simulink model "flightControlSystem"  (R2024b)
settings: Solver=ode3  StartTime=0  StopTime=TFinal  FixedStep=Ts  RelTol=1e-3  EnableMultiTasking=on
undefined symbols (not defined in the file): BINARIZER_THRESHOLD, codertarget, COG_X, COG_Xe, COG_Y, COG_Ye, Controller, DELAY_LANDING, DERIVATIVE_GAIN_X, DERIVATIVE_GAIN_Y, DiscIntNeverNeededParam, Discrete, DISK_KERNEL, Estimator, FLAG_WAIT_FOR_HOVERING, FOV, FOV_inner, FRAME_SIZE_HEIGHT, FRAME_SIZE_WIDTH, g, GAIN_LANDING, GAIN_TRACK, gray, init, MAX_RADIUS_CROWN, MAX_RADIUS_TRACK, MIN_RADIUS_CROWN, MIN_RADIUS_TRACK, Sensors, SQUARE_KERNEL, strel, Time, TIME_HOLD_X, TIME_HOLD_Y, Ts, var_acc_angle_N, var_bias_gyr_N, var_gyro_p_N, Vehicle, Z_HIGH, Z_LOW
libraries: simulink x39, slpidlib x4, ctrlSharedLib x4, sharedtransform x3, visionmorphops x2, parrotlib x1
(part 3 of 3)

== matlab function flightControlSystem/Image Processing System/MATLAB Function1 ==
  data: binary input; error_x_end_marker output; waypoint_follower_variable input; FRAME_SIZE_WIDTH input; FRAME_SIZE_HEIGHT input; COG_Y input; COG_X input; error_y_end_marker output; flag_end_marker output
function [error_x_end_marker, error_y_end_marker, flag_end_marker] = end_marker_detector(binary, waypoint_follower_variable, ...
    FRAME_SIZE_WIDTH, FRAME_SIZE_HEIGHT, COG_Y, COG_X)


persistent column_accumulator
persistent count_pixel
persistent row_accumulator

if isempty(column_accumulator)
    column_accumulator = 0;
end

if isempty(count_pixel)
    count_pixel = 0;
end

if isempty(row_accumulator)
    row_accumulator = 0;
end

flag_track = waypoint_follower_variable(3);

% check if the track is ended
if ~flag_track

    for i=1:FRAME_SIZE_HEIGHT

        for j=1:FRAME_SIZE_WIDTH

            %check all the pixel belonging to the end marker
            if binary(i,j)==1
                count_pixel = count_pixel +1;
                column_accumulator = column_accumulator + j;
                row_accumulator = row_accumulator + i;

            end

        end
    end
    
    if count_pixel ~= 0
        flag_end_marker=1;
        center_x = round(row_accumulator/count_pixel);
        center_y = round(column_accumulator/count_pixel);
    else
        flag_end_marker=0;              %for last push to the landing location
        center_x=0;
        center_y=0;
    end

else
    
    center_x = 0;
    center_y = 0;
    flag_end_marker = 0;

end

% Calculate the medium point of the end marker
error_x_end_marker = -(center_x - COG_X);
error_y_end_marker = (center_y - COG_Y);

% reset of the persistent variables
count_pixel = 0;
column_accumulator = 0;
row_accumulator = 0;

end

== stateflow chart flightControlSystem/Control System/Path Planning/Chart ==
  state State0
    during:
    x_error = 0;
    y_error = 0;
  state State2
    during:
    x_error = x_err_tr;
    y_error = y_err_tr;
  state State3
    during:
    x_error = x_err_ea;
    y_error = y_err_ea;
  State3 -> State0 [order 2] : [flag_ho ~= 1]
  (default) -> State0
  State0 -> State2 [order 1] : [flag_ho == 1 && flag_ea == 0]
  State2 -> State3 [order 1] : [flag_ho == 1 && flag_ea ~= 0]
  State3 -> State2 [order 1] : [flag_ho == 1 && flag_ea == 0]
  State2 -> State0 [order 2] : [flag_ho ~= 1]
  State0 -> State3 [order 2] : [flag_ho == 1 && flag_ea ~= 0]
  data: x_err_tr input; y_err_tr input; x_err_ea input; y_err_ea input; flag_ea input; flag_ho input; x_error output; y_error output

== stateflow chart flightControlSystem/Control System/Path Planning/Take off Checker ==
  state state0
    entry: flag_activate_PP = 0 ;
  state state1
    entry: flag_activate_PP = 0 ;
  state state2
    entry: flag_activate_PP = 1 ;
  (default) -> state0
  state0 -> state1 [order 1] : [FLAG_WAIT_FOR_HOVERING == 0]
  state1 -> state2 : [z_est < Z_LOW && z_est > Z_HIGH]
  state2 -> state1 : [z_est > Z_LOW || z_est < Z_HIGH]
  state0 -> state2 [order 2] : [FLAG_WAIT_FOR_HOVERING == 1]
  data: z_est input; flag_activate_PP output; FLAG_WAIT_FOR_HOVERING parameter; Z_HIGH parameter; Z_LOW parameter

== matlab function flightControlSystem/Control System/Path Planning/Non linear Path Planner/X_PLANNER/x_derivative_contribute /derivative error ==
  data: dev_contribute_prev input; derivative_error input; flag_change_error input; dev_contribute output; count_prev input; count output; flag_count_prev input; flag_count output; Ts parameter; TIME_HOLD_X parameter; DERIVATIVE_GAIN_X parameter
function [dev_contribute, count, flag_count] = derivative_error(dev_contribute_prev, ...
    derivative_error, flag_change_error,count_prev,flag_count_prev, Ts, ...
    TIME_HOLD_X, DERIVATIVE_GAIN_X)

persistent count_to_be_hold

if isempty(count_to_be_hold)
    count_to_be_hold = round(TIME_HOLD_X/Ts);
end

flag_count = 0;

if flag_change_error && count_prev == 0    
    flag_count=1;   
end
   
if flag_count_prev || flag_count
    
    if count_prev == count_to_be_hold

        count=0;
        flag_count=0;

    else

        count=count_prev+1;
        flag_count=1;
        
    end
    
    dev_contribute=derivative_error*DERIVATIVE_GAIN_X;
    
    if dev_contribute ==0 && dev_contribute_prev ~=0 
        
        dev_contribute=dev_contribute_prev;
        
    end

else
    
    flag_count = 0;
    count = 0;
    dev_contribute = 0;
    
end

== matlab function flightControlSystem/Control System/Path Planning/Non linear Path Planner/Y_PLANNER/y_derivative_contribute /MATLAB Function ==
  data: derivative_error input; flag_change_error output; CHANGE_DERIVATIVE_ERROR_THRESHOLD_Y parameter
function flag_change_error = change_error_checker(derivative_error, ...
    CHANGE_DERIVATIVE_ERROR_THRESHOLD_Y)

if abs(derivative_error) >= CHANGE_DERIVATIVE_ERROR_THRESHOLD_Y

    flag_change_error = 1;

else

    flag_change_error = 0;

end

== stateflow chart flightControlSystem/Control System/Path Planning/Non linear Path Planner/Z PLANNER/Chart ==
  state STATE [group]
    - TRACKING: The drone is tracking the lane or the end-marker when they are detected.
    - LANDING: The drone is landing when the land-marker is detected and the error between the drone CoG and
    the central point of the end-marker is less than MAX_ERROR_LANDING.
  state INPUT [group]
    - flag_track: flag raised when the lane is detected by the Image Processing System.
    - flag_end_marker: flag raised when the end-marker is detected by the Image Processing System.
    - norm error: error between the drone CoG and the central point of the end-marker.
  state OUTPUT [group]
    - z_planned: drone altitude sent to the drone controller.
    - flag_end_marker_to_controller: flag raise when the drone has to land.
  state TRACKING
    entry:
    z_planned =  -1.1 ;
    flag_end_marker_to_controller=0;
  state IDLE
    entry:
    z_planned =  -1.1 ;
    flag_end_marker_to_controller=0;
  state LANDING_START
    during:
    z_planned = z_planned + 0.001 ;
    flag_end_marker_to_controller=1;
  state LANDING_STOP
    entry:
    z_planned = 0 ;
    flag_end_marker_to_controller=1;
  (default) -> IDLE
  IDLE -> TRACKING : [flag_track==1]
  TRACKING -> LANDING_START : [flag_end_marker==1 && norm_error <= MAX_ERROR_LANDING]
  LANDING_START -> LANDING_STOP : [z_planned >= -0.15]
  data: norm_error input double; z_planned output double; MAX_ERROR_LANDING parameter double; flag_end_marker input; flag_track input; flag_end_marker_to_controller output double

== stateflow chart flightControlSystem/Control System/Path Planning/Non linear Path Planner/X_PLANNER/x_linear_contribute ==
  state STATE [group]
    - TRACK_DETECTED: The Image Processing System detected the lane.
    - END_MARKER_DETECTED: The Image Processing System detected the end-marker.
  state INPUT [group]
    - Flag_track: flag raised when the lane is detected by the Image Processing System.
    - Flag_end_marker : flag raised when the end-marker is detected by the Image Processing System.
  state PARAMETERS [group]
    - GAIN_TRACK: gain used from the drone reference generator when it follows the lane.
    - GAIN_LANDING: gain used from the drone reference generator for landing on the end-marker.
  state OUTPUT [group]
    - linear_part : linear contribute.
  state END_MARKER_DETECTED
    during:
    linear_part = error * GAIN_LANDING;
  state IDLE
  state TRACK_DETECTED
    during:
    linear_part = error * GAIN_TRACK;
  TRACK_DETECTED -> END_MARKER_DETECTED : [flag_end_marker==1 && flag_track==0]
  IDLE -> TRACK_DETECTED : [flag_end_marker==0 && flag_track==1]
  (default) -> IDLE
  data: error input double; GAIN_TRACK parameter double; GAIN_LANDING parameter double; flag_end_marker input double; flag_track input double; linear_part output double

== matlab function flightControlSystem/Control System/Path Planning/Non linear Path Planner/Z PLANNER/MATLAB Function ==
  data: norm_error_tot output; error_x input; norm_error output; error_y input; flag_end_marker input; norm_error_prev input
function [norm_error_tot, norm_error] = error_function(error_x, error_y, ...
flag_end_marker, norm_error_prev)

if flag_end_marker
    
    norm_error = sqrt((error_x)^2 + (error_y)^2);
    norm_error_tot = norm_error + norm_error_prev  ;
    
else 
    %100 is a constant value greater than MAX_ERROR_LANDING
    norm_error_tot = 100;
    norm_error = 100;
end

== matlab function flightControlSystem/Control System/Path Planning/Non linear Path Planner/Y_PLANNER/y_derivative_contribute /derivative error ==
  data: dev_contribute_prev input; derivative_error input; flag_change_error input; dev_contribute output; count_prev input; count output; flag_count_prev input; flag_count output; Ts parameter; TIME_HOLD_Y parameter; DERIVATIVE_GAIN_Y parameter
function [dev_contribute, count, flag_count] = derivative_error(dev_contribute_prev, ...
    derivative_error, flag_change_error,count_prev,flag_count_prev, Ts, ...
    TIME_HOLD_Y, DERIVATIVE_GAIN_Y)

persistent count_to_be_hold

if isempty(count_to_be_hold)
    count_to_be_hold = round(TIME_HOLD_Y/Ts);
end

flag_count = 0;

if flag_change_error && count_prev == 0    
    flag_count=1;   
end
   
if flag_count_prev || flag_count
    
    if count_prev == count_to_be_hold

        count=0;
        flag_count=0;

    else

        count=count_prev+1;
        flag_count=1;
        
    end
    
    dev_contribute=derivative_error*DERIVATIVE_GAIN_Y;
    
    if dev_contribute ==0 && dev_contribute_prev ~=0 
        
        dev_contribute=dev_contribute_prev;
        
    end

else
    
    flag_count = 0;
    count = 0;
    dev_contribute = 0;
    
end

== matlab function flightControlSystem/Control System/Path Planning/Non linear Path Planner/X_PLANNER/x_derivative_contribute /MATLAB Function ==
  data: derivative_error input; flag_change_error output; CHANGE_DERIVATIVE_ERROR_THRESHOLD_X parameter
function flag_change_error = change_error_checker(derivative_error, ...
    CHANGE_DERIVATIVE_ERROR_THRESHOLD_X)

if abs(derivative_error) >= CHANGE_DERIVATIVE_ERROR_THRESHOLD_X

    flag_change_error = 1;

else

    flag_change_error = 0;

end

== stateflow chart flightControlSystem/Control System/Path Planning/Non linear Path Planner/Y_PLANNER/Chart1 ==
  state STATE [group]
    - TRACKING: the drone is tracking the lane of the end-marker.
    - LANDING: the drone is landing when the end-marker is dected and the error between the drone CoG and the
    middle point of the end-marker is less than MAX_ERROR_LANDING.
    - TRACK_DETECTED: the Image Processing System detected the lane.
    - END_MARKER_DETECTED: the Image Processing System detected the end-marker.
  state INPUT [group]
    - flag_track: flag raised when the track is detected by Image Processing System.
    - flag_end_marker_to_Controller: flag raised when the drone has to land.
    - lin_part: linear part of the path planner.
    - dev_part: derivative part of the path planner.
    - y_estimated: estimated drone position along the y-axis.
    - flag_end_marker : flag raised when the end-marker is detected by the Image Processing System.
  state OUTPUT [group]
    - y_planned: y coordinate of the goal position.
  state TRACKING
    state TRACK_DETECTED
      during:
      y_planned= y_estimated + lin_part + dev_part;
      y_planned_stored=y_planned;
    state END_MARKER_DETECTED
      during:
      y_planned= y_estimated + lin_part ;
      y_planned_stored=y_planned;
    (default) -> TRACK_DETECTED
    TRACK_DETECTED -> END_MARKER_DETECTED : [flag_end_marker==1 && flag_track==0]
    END_MARKER_DETECTED -> TRACK_DETECTED : [flag_end_marker==0 && flag_track==1]
  state LANDING
    during:
    y_planned=y_planned_stored;
  state IDLE
  (default) -> IDLE
  IDLE -> TRACKING : [flag_track==1 && flag_end_marker==0]
  TRACKING -> LANDING : [flag_end_marker_to_controller==1]
  data: dev_part input double; lin_part input double; flag_end_marker_to_controller input double; flag_track input double; flag_end_marker input double; y_estimated input; y_planned_stored local double; y_planned output double

== stateflow chart flightControlSystem/Control System/Path Planning/Non linear Path Planner/X_PLANNER/Chart1 ==
  state STATE [group]
    - TRACKING: The drone is tracking the lane or the end-marker.
    - LANDING: The drone is landing if the end-marker is detected and the error between the drone CoG and the middle
    point of the end-marker is less than MAX_ERROR_LANDING.
    - TRACK_DETECTED: The Image Processing System detected the lane.
    - END_MARKER_DETECTED: The Image Processing System detected the end-marker.
  state INPUT [group]
    - flag_track: flag raised when the track is detected by the Image Processing System.
    - flag_end_marker_to_controller: flag raised when the drone has to land.
    - lin_part: linear part of the path planner.
    - dev_part: derivative part of the path planner.
    - x_estimated: postion x estimated from the sensors.
    - flag_end_marker: flag raised when the land-marker is detected by the Image Processing System.
  state OUTPUT [group]
    - x_planned: x coordinate of the goal position.
  state TRACKING
    state TRACK_DETECTED
      during:
      x_planned = x_estimated + lin_part + dev_part;
      x_planned_stored = x_planned;
    state END_MARKER_DETECTED
      during:
      x_planned = x_estimated + lin_part ;
      x_planned_stored = x_planned;
    (default) -> TRACK_DETECTED
    TRACK_DETECTED -> END_MARKER_DETECTED : [flag_end_marker==1 && flag_track==0]
    END_MARKER_DETECTED -> TRACK_DETECTED : [flag_end_marker==0 && flag_track==1]
  state LANDING
    during:
    x_planned=x_planned_stored;
  state IDLE
  (default) -> IDLE
  IDLE -> TRACKING : [flag_track==1 && flag_end_marker==0]
  TRACKING -> LANDING : [flag_end_marker_to_controller==1]
  data: dev_part input double; lin_part input double; x_planned output double; flag_end_marker_to_controller input double; x_estimated input double; flag_track input double; x_planned_stored local double; flag_end_marker input double

== stateflow chart flightControlSystem/Control System/Path Planning/Non linear Path Planner/Y_PLANNER/y_linear_contribute ==
  state STATE [group]
    - TRACKING: the drone is tracking the lane or the end-marker.
    - LANDING: the drone lands when the end-marker is detected and the error between the drone CoG and the middle
    of the end-marker is less than MAX_ERROR_LANDING.
    - TRACK_DETECTED: the Image Processing System detected the lane.
    - END_MARKER_DETECTED: the Image Processing System detected the end-marker.
  state INPUT [group]
    - flag_track: flag raised when the lane is detected by Image Processing System.
    - flag_end_marker_to_controller: flag raised when the drone has to land.
    - lin_part: linear part of the path planner.
    - dev_part: derivative part of the path planner.
    - y_estimated: y coordinate of the drone position.
    - flag_end_marker: flag raised when the end-marker is detected by Image Processing System.
  state PARAMETERS [group]
    - GAIN_TRACK: gain used by the drone reference generator to follow the lane.
    - GAIN_LANDING: gain used by the drone reference generator to land over the end-marker.
  state OUTPUT [group]
    - y_planned: y coordinate of the goal position.
  state END_MARKER_DETECTED
    during:
    linear_part = error * GAIN_LANDING;
  state IDLE
  state TRACK_DETECTED
    during:
    linear_part = error * GAIN_TRACK;
  TRACK_DETECTED -> END_MARKER_DETECTED : [flag_end_marker==1 && flag_track==0]
  IDLE -> TRACK_DETECTED : [flag_end_marker==0 && flag_track==1]
  (default) -> IDLE
  data: error input double; GAIN_TRACK parameter double; GAIN_LANDING parameter double; flag_end_marker input double; flag_track input double; linear_part output double

== stateflow chart flightControlSystem/Image Processing System/state machine1 ==
  state STATE [group]
    - ON_TRACK: the Image Processing System detects the lane. The drone is on the lane.
    - END_TRACK: it indicates the end of the lane.
  state OUTPUT [group]
    - FLAG: it indicates the presence or not of the track path
  state INPUT [group]
    - FLAG_TRACK: flag raises when the track is detected from Image Processing System.
  state END_TRACK
    entry: flag=0;
  state ON_TRACK
    entry: flag=1;
  state delay
    entry:
    flag=1;
  state TAKE_OFF
    entry: flag=1;
  ON_TRACK -> END_TRACK : [flag_track==0]
  delay -> ON_TRACK : [flag_track==1]
  (default) -> TAKE_OFF
  TAKE_OFF -> delay : after(1,sec)
  END_TRACK -> ON_TRACK : [A == 0]
  data: A input; flag output; flag_track input

== matlab function flightControlSystem/Image Processing System/MATLAB Function ==
  data: frame input; error_y_track output; x_ref_prev input; y_ref_prev input; flag_track_prev input; MIN_RADIUS_CROWN input; MAX_RADIUS_CROWN input; error_x_track output; orientation_track output; flag_track output; img2 output; MIN_RADIUS_TRACK input; MAX_RADIUS_TRACK input; FOV input; FOV_inner input; COG_X input; COG_Y input; angle_between_headings output; outer_side_flag output; fork_detect output
function [error_y_track, error_x_track, orientation_track, flag_track, img2, angle_between_headings, outer_side_flag, fork_detect] = ...
    error_pixel_generator(frame, x_ref_prev, y_ref_prev, flag_track_prev, ...
    MIN_RADIUS_CROWN, MAX_RADIUS_CROWN, MIN_RADIUS_TRACK, MAX_RADIUS_TRACK, ...
    FOV,FOV_inner, COG_X, COG_Y)
% ==========================================================
% FUNCTION: error_pixel_generator
%
% PURPOSE:
%   - Detect lane center within two crown-shaped masks:
%       1. Inner crown (inner lane region)
%       2. Outer crown (outer lane region / track)
%   - Compute tracking errors based on detected lane positions.
%   - Visualize lane points, center of gravity, and FOV boundaries.
%
% OUTPUTS:
%   error_y_track          : Lateral pixel error in Y direction for inner crown
%   error_x_track          : Lateral pixel error in X direction for inner crown
%   orientation_track      : Heading angle of lane based on previous reference
%   flag_track             : True if valid lane points were detected
%   img2                   : Visualization image with markings
%   angle_between_headings : Angle between inner & outer VTP headings
%   outer_side_flag        : Indicates which side outer VTP lies (+1 left, -1 right, 0 aligned)
%
% NOTE:
%   - Uses persistent accumulators for pixel detection.
% ==========================================================


%% ==========================================================
% 1. PERSISTENT VARIABLES INITIALIZATION
% ==========================================================
    persistent x_accumulator y_accumulator pixel_count heading_angle_inner heading_angle_outer  
    persistent fork_value fork_timer


    if isempty(x_accumulator), x_accumulator = 0; end
    if isempty(y_accumulator), y_accumulator = 0; end
    if isempty(pixel_count), pixel_count = 0; end
    if isempty(heading_angle_inner), heading_angle_inner = 0; end
    if isempty(heading_angle_outer), heading_angle_outer = 0; end
    if isempty(fork_value), fork_value = 0; end
    if isempty(fork_timer), fork_timer = 0; end

% Default outputs to safe values
    angle_between_headings = 0;   % Angle difference between inner and outer headings
    outer_side_flag = 0;          % Default = aligned

% Frame dimensions
    rows = size(frame,1);
    columns = size(frame,2);


%% ==========================================================
% 2. FRAME PREPARATION (RGB & GRAYSCALE)
% ==========================================================
% Convert grayscale to RGB for visualization
    if size(frame,3) == 1
        img2 = repmat(frame, [1 1 3]);
    else
        img2 = frame;
    end
    
    % Keep a grayscale version for detection
    grayFrame = frame;
    if size(frame,3) == 3
        grayFrame = rgb2gray(frame);
    end


%% ==========================================================
% 3. ORIENTATION & FIELD OF VIEW (FOV) LIMITS
% ==========================================================
% Previous lane orientation based on last reference point
    orientation_track = atan2(-x_ref_prev, y_ref_prev);
    orientation_track = mod(orientation_track, 2*pi);
    
    % Define angular thresholds for the detection FOV
    threshold_1 = mod((orientation_track + (pi/FOV)), 2*pi);
    threshold_2 = mod((orientation_track - (pi/FOV)), 2*pi);
    threshold_1_inner = mod((orientation_track + (pi/FOV_inner)), 2*pi);
    threshold_2_inner = mod((orientation_track - (pi/FOV_inner)), 2*pi);

%% ==========================================================
% 4. INNER CROWN DETECTION (Virtual Target Point - VTP)
% ==========================================================
    if flag_track_prev
        % --- With FOV restriction ---


        for i = (COG_X - MAX_RADIUS_CROWN):(COG_X + MAX_RADIUS_CROWN)
            for j = (COG_Y - MAX_RADIUS_CROWN):(COG_Y + MAX_RADIUS_CROWN)
    
                % Ignore pixels outside frame
                if i<1 || j<1 || i>rows || j>columns, continue; end
    
                % Radial distance from COG
                norm_val = sqrt(((i-(COG_X-0.5))^2) + ((j-(COG_Y-0.5))^2));
    
                % Within inner crown radius
                if norm_val >= MIN_RADIUS_CROWN && norm_val <= MAX_RADIUS_CROWN
                    % Compute angle to pixel
                    axis_x = (i-(COG_X-0.5));
                    axis_y = (j-(COG_Y-0.5));
                    yaw_point_temp_2 = mod(atan2(axis_x, axis_y), 2*pi);
    
                    % Check if within FOV arc
                    if threshold_1 < threshold_2
                        flag_threshold = ...
                            (yaw_point_temp_2 <= 2*pi && yaw_point_temp_2 >= threshold_2) ...
                            || (yaw_point_temp_2 <= threshold_1 && yaw_point_temp_2 >= 0);
                    else
                        flag_threshold = yaw_point_temp_2 <= threshold_1 && yaw_point_temp_2 >= threshold_2;
                    end
    
                    % If pixel is lane (value=1), accumulate for averaging
                    if flag_threshold && grayFrame(i,j) == 1
                        pixel_count = pixel_count + 1;
                        x_accumulator = x_accumulator + i;
                        y_accumulator = y_accumulator + j;
                    end
                end
            end
        end
    else
        % --- Without FOV restriction (first detection) ---

        for i = (COG_X - MAX_RADIUS_CROWN):(COG_X + MAX_RADIUS_CROWN)
            for j = (COG_Y - MAX_RADIUS_CROWN):(COG_Y + MAX_RADIUS_CROWN)
    
                if i<1 || j<1 || i>rows || j>columns, continue; end
                norm_val = sqrt(((i-(COG_X-0.5))^2) + ((j-(COG_Y-0.5))^2));
    
                if norm_val >= MIN_RADIUS_CROWN && norm_val <= MAX_RADIUS_CROWN
                    if grayFrame(i,j) == 1
                        pixel_count = pixel_count + 1;
                        x_accumulator = x_accumulator + i;
                        y_accumulator = y_accumulator + j;
                    end
                end
            end
        end
        % Horizontal case only
        % if Left-up , Right-up : + 250 ; if left-down , Right-down : - 250
        x_accumulator = x_accumulator + 250;
        % Vertical case ignored now
        %y_accumulator = y_accumulator - 500;
    end


%% ==========================================================
% 5. INNER ERROR CALCULATION (Center of detected pixels)
% ==========================================================
    if pixel_count > 0
        % Centroid of detected pixels
        cx = round(x_accumulator / pixel_count);
        cy = round(y_accumulator / pixel_count);
    
        % Pixel errors relative to COG
        x_ref_temp = -(cx - COG_X);
        y_ref_temp =  (cy - COG_Y);
    
        error_x_track = x_ref_temp;
        error_y_track = y_ref_temp;
    
        flag_error_x = true;
        flag_error_y = true;
    else
        % No detection -> zero error
        cx = COG_X;
        cy = COG_Y;
        error_x_track = 0;
        error_y_track = 0;
        flag_error_x = false;
        flag_error_y = false;
    end

% Detection flag
    flag_track = flag_error_x || flag_error_y;


%% ==========================================================
% 6. OUTER CROWN (TRACK) DETECTION
% ==========================================================
    track_x_accum = 0;
    track_y_accum = 0;
    track_pixel_count = 0;
    
    if flag_track_prev
        % --- With FOV restriction ---

        for i = (COG_X - MAX_RADIUS_TRACK):(COG_X + MAX_RADIUS_TRACK)
            for j = (COG_Y - MAX_RADIUS_TRACK):(COG_Y + MAX_RADIUS_TRACK)
    
                if i<1 || j<1 || i>rows || j>columns, continue; end
                norm_val = sqrt(((i-(COG_X-0.5))^2) + ((j-(COG_Y-0.5))^2));
    
                if norm_val >= MIN_RADIUS_TRACK && norm_val <= MAX_RADIUS_TRACK
                    axis_x = (i-(COG_X-0.5));
                    axis_y = (j-(COG_Y-0.5));
                    yaw_point_temp_2 = mod(atan2(axis_x, axis_y), 2*pi);
    
                    if threshold_1_inner < threshold_2_inner
                        flag_threshold = ...
                            (yaw_point_temp_2 <= 2*pi && yaw_point_temp_2 >= threshold_2_inner) ...
                            || (yaw_point_temp_2 <= threshold_1_inner && yaw_point_temp_2 >= 0);
                    else
                        flag_threshold = yaw_point_temp_2 <= threshold_1_inner && yaw_point_temp_2 >= threshold_2_inner;
                    end
    
                    if flag_threshold && grayFrame(i,j) == 1
                        track_pixel_count = track_pixel_count + 1;
                        track_x_accum = track_x_accum + i;
                        track_y_accum = track_y_accum + j;
                    end
                end
            end
        end
    else
        % --- Without FOV restriction ---

        for i = (COG_X - MAX_RADIUS_TRACK):(COG_X + MAX_RADIUS_TRACK)
            for j = (COG_Y - MAX_RADIUS_TRACK):(COG_Y + MAX_RADIUS_TRACK)
    
                if i<1 || j<1 || i>rows || j>columns, continue; end
                norm_val = sqrt(((i-(COG_X-0.5))^2) + ((j-(COG_Y-0.5))^2));
    
                if norm_val >= MIN_RADIUS_TRACK && norm_val <= MAX_RADIUS_TRACK
                    if grayFrame(i,j) == 1
                        track_pixel_count = track_pixel_count + 1;
                        track_x_accum = track_x_accum + i;
                        track_y_accum = track_y_accum + j;
                    end
                end
            end
        end
    end
    
    % Centroid for outer VTP
    if track_pixel_count > 0
        cx_track = round(track_x_accum / track_pixel_count);
        cy_track = round(track_y_accum / track_pixel_count);
        flag_track_vtp = true;
    else
        cx_track = COG_X;
        cy_track = COG_Y;
        flag_track_vtp = false;
    end



%% ==========================================================
% 7. VISUALIZATION (COG, Crowns, VTPs, FOV Arcs)
% ==========================================================
% Draw COG (black square)
    for dx = -1:1
        for dy = -1:1
            xi = COG_X + dx;
            yj = COG_Y + dy;
            if xi>0 && yj>0 && xi<=rows && yj<=columns
                img2(xi,yj,:) = uint8([0 0 0]);
            end
        end
    end

% Draw inner crown boundaries (red)
    theta_vals = linspace(0, 2*pi, 360);
    for r_val = [MIN_RADIUS_CROWN, MAX_RADIUS_CROWN]
        for t = theta_vals
            xi = round(COG_X + r_val * cos(t));
            yj = round(COG_Y + r_val * sin(t));
            if xi > 0 && yj > 0 && xi <= rows && yj <= columns
                img2(xi, yj, :) = uint8([255 0 0]);
            end
        end
    end

% Draw outer track boundaries (green)
    for r_val = [MIN_RADIUS_TRACK, MAX_RADIUS_TRACK]
        for t = theta_vals
            xi = round(COG_X + r_val * cos(t));
            yj = round(COG_Y + r_val * sin(t));
            if xi > 0 && yj > 0 && xi <= rows && yj <= columns
                img2(xi, yj, :) = uint8([0 255 0]);
            end
        end
    end

% Half FOV in radians
    half_fov_rad = FOV / 2;
    half_fov_rad_inner = FOV_inner/2;

% ---- Draw Inner VTP ----
    if pixel_count > 0
        % Mark point (black)
        for dx = -1:1
            for dy = -1:1
                xi = cx + dx;
                yj = cy + dy;
                if xi>0 && yj>0 && xi<=rows && yj<=columns
                    img2(xi,yj,:) = uint8([0 0 0]);
                end
            end
        end
    
        % Heading line (black)
        heading_angle_inner = atan2(cy - COG_Y, cx - COG_X);
        img2 = bresenhamLine(img2, COG_X, COG_Y, cx, cy, [0 0 0]);
    
        % FOV boundaries (blue)
        arrow_length_inner = sqrt((cx - COG_X)^2 + (cy - COG_Y)^2);
        img2 = bresenhamLine(img2, COG_X, COG_Y, ...
            round(COG_X + arrow_length_inner * cos(heading_angle_inner + half_fov_rad)), ...
            round(COG_Y + arrow_length_inner * sin(heading_angle_inner + half_fov_rad)), ...
            [0 0 255]);
        img2 = bresenhamLine(img2, COG_X, COG_Y, ...
            round(COG_X + arrow_length_inner * cos(heading_angle_inner - half_fov_rad)), ...
            round(COG_Y + arrow_length_inner * sin(heading_angle_inner - half_fov_rad)), ...
            [0 0 255]);
    end

% ---- Draw Outer VTP ----
    if flag_track_vtp
        for dx = -1:1
            for dy = -1:1
                xi = cx_track + dx;
                yj = cy_track + dy;
                if xi>0 && yj>0 && xi<=rows && yj<=columns
                    img2(xi,yj,:) = uint8([255 0 255]);
                end
            end
        end
    
        heading_angle_outer = atan2(cy_track - COG_Y, cx_track - COG_X);
        img2 = bresenhamLine(img2, COG_X, COG_Y, cx_track, cy_track, [255 0 255]);
    
        arrow_length_outer = sqrt((cx_track - COG_X)^2 + (cy_track - COG_Y)^2);
        img2 = bresenhamLine(img2, COG_X, COG_Y, ...
            round(COG_X + arrow_length_outer * cos(heading_angle_outer + half_fov_rad_inner)), ...
            round(COG_Y + arrow_length_outer * sin(heading_angle_outer + half_fov_rad_inner)), ...
            [0 255 255]);
        img2 = bresenhamLine(img2, COG_X, COG_Y, ...
            round(COG_X + arrow_length_outer * cos(heading_angle_outer - half_fov_rad_inner)), ...
            round(COG_Y + arrow_length_outer * sin(heading_angle_outer - half_fov_rad_inner)), ...
            [0 255 255]);
    end



%% ==========================================================
% 8. RESET FOR NEXT FRAME
% ==========================================================
pixel_count = 0;
x_accumulator = 0;
y_accumulator = 0;

    function img = bresenhamLine(img, x1, y1, x2, y2, color)
        dx = abs(x2 - x1);
        dy = abs(y2 - y1);
        sx = sign(x2 - x1);
        sy = sign(y2 - y1);
        err = dx - dy;
    
        while true
            if x1 > 0 && y1 > 0 && x1 <= size(img,1) && y1 <= size(img,2)
                img(x1, y1, :) = uint8(color);
            end
            if x1 == x2 && y1 == y2
                break;
            end
            e2 = 2 * err;
            if e2 > -dy
                err = err - dy;
                x1 = x1 + sx;
            end
            if e2 < dx
                err = err + dx;
                y1 = y1 + sy;
            end
        end
    end

    %% ==========================================================
    % 9. ANGLE BETWEEN HEADINGS
    % ==========================================================
    % Ensure both headings were calculated before proceeding.
    % Calculate the signed angle difference. The order (inner - outer) ensures
    % a positive result when the outer heading is to the right (clockwise).
    angle_between_headings = atan2(sin(heading_angle_inner - heading_angle_outer), cos(heading_angle_inner - heading_angle_outer))*180/pi;%in degree

    % Determine the side flag based on the angle's sign.
    % +1 = Left (angle is negative)
    % -1 = Right (angle is positive)
    % 0 = Aligned (angle is zero)
    if angle_between_headings > 10
        outer_side_flag = -1;
    elseif angle_between_headings < -10
        outer_side_flag = 1;
    else
        outer_side_flag = 0;
    end
    %% ==========================================================
    % 10. FORK DETECTION
    % ==========================================================
    if isempty(fork_value)
        fork_value = 0; 
        fork_timer = 0;
    end
    
    if  fork_value == 0 && outer_side_flag ~= 0
        % First non-zero detection while fork_flag is active
        fork_value = outer_side_flag;
        fork_timer = 5; % seconds to hold
    end
    
    % If we're holding a value, countdown the timer
    if fork_timer > 0
        fork_timer = fork_timer - 0.0333; % Ts in seconds
        if fork_timer <= 0
            fork_value = 0; % reset after time expires
        end
    end
    
    fork_detect = fork_value;

end
